simulink model "RollingMill_PLC"  (R2020b)
settings: Solver=ode1be  StartTime=0.0  StopTime=inf  RelTol=1e-3
values from neighbouring files (symbols this model uses):
  sysd_2 = c2d(sysc,0.01)    [Rolling_mill_matlab.m]
libraries: simulink x4, opclib x1
settings Model: Creator=Mehrab  LastModifiedBy=Mehrab
settings DataIOCC: LimitDataPoints=on  SaveFormat=Array  SaveOutput=off  SaveTime=off
settings OptimizationCC: LifeSpan=1
settings HardwareCC: ProdBitPerPointer=32  ProdBitPerSizeT=32  ProdBitPerPtrDiffT=32  ProdWordSize=32  ProdHWDeviceType=Intel->x86-32 (Windows32)
settings RTWCC: Description=Target for ODK capable S7-1500 Controllers based on Simulink Coder  SystemTargetFile=Target_1500S_V4_0_grt.tlc  GenCodeOnly=on  GenerateMakefile=off  TemplateMakefile=Target_1500S_V4_0_grt.tmf  RTWVerbose=off  TargetLang=C++
settings CodeAppCC: MaxIdLength=256
settings STFCustomTargetCC: TargetLangStandard=C++03 (ISO)  ParMdlRefBuildCompliant=on  ConcurrentExecutionCompliant=off  CombineOutputUpdateFcns=on  CPPClassGenCompliant=off  GRTInterface=off  SystemTargetFile=Target_1500S_V4_0_grt.tlc
settings GRTTargetCC: TargetLangStandard=C++03 (ISO)  CompOptLevelCompliant=off  ConcurrentExecutionCompliant=off  MatFileLogging=off  CPPClassGenCompliant=off  UseToolchainInfoCompliant=off  ExtModeStaticAlloc=on  ExtModeMexFile=mwsl_ii_ext_comm_target1500s_v4  ExtModeMexArgs='192.168.3.3' 0 17725 0

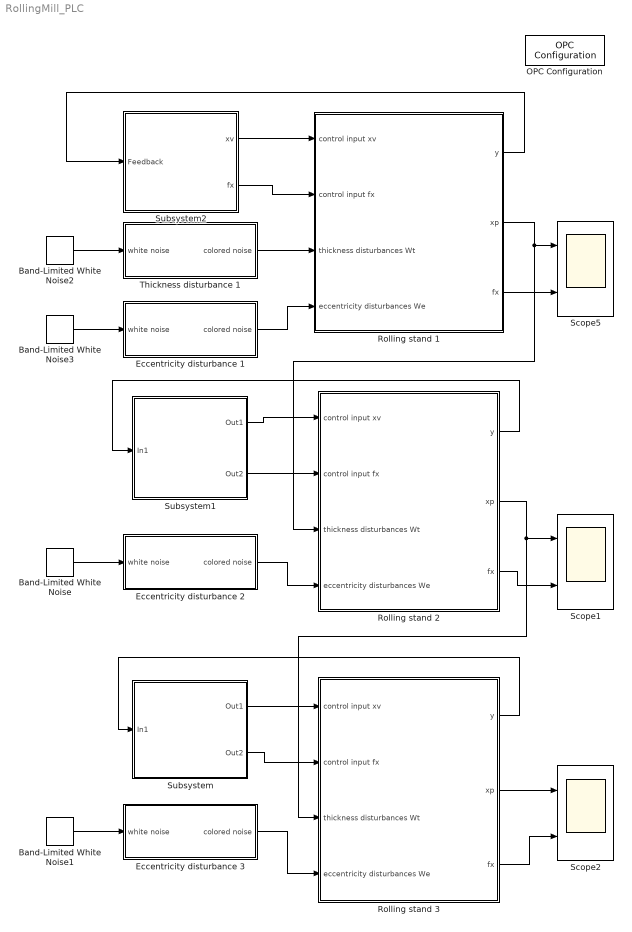
== system RollingMill_PLC ==
  Band-Limited White Noise : simulink/Sources/Band-Limited White Noise  Cov=[0.0001]  Ts=0.01  seed=[21241]
  Band-Limited White Noise1 : simulink/Sources/Band-Limited White Noise  Cov=[0.00001]  Ts=0.01  seed=[63341]
  Band-Limited White Noise2 : simulink/Sources/Band-Limited White Noise  Cov=[15]  Ts=0.01  seed=[23341]
  Band-Limited White Noise3 : simulink/Sources/Band-Limited White Noise  Cov=[0.0001]  Ts=0.01  seed=[65441]
  Eccentricity disturbance 1 : Subsystem
  Eccentricity disturbance 2 : Subsystem
  Eccentricity disturbance 3 : Subsystem
  OPC Configuration : opclib/OPC Configuration  errMissingItems=Error  errReadWrite=Warn  errShutdown=Error  errRTViolation=Warn  rtEnable=on  speedup=1  showLatency=off  beingUsed=on
      settings: SourceProductBaseCode=OT
  Rolling stand 1 : Subsystem
      mask Display:
      | image('$imagefile'); % Use "Edit Image" on toolstrip to change.
      | color('blue');port_label('input', 1, 'xv');
      | port_label('input', 2, 'fx');
      | color('red');port_label('input', 3, 'Wt');
      | port_label('input', 4, 'We');
      | color('black');port_label('output', 1, 'y');
      | port_label('output', 2, 'xp');
      | port_label('output', 3, 'fx');
  Rolling stand 2 : Subsystem
      mask Display:
      | image('$imagefile'); % Use "Edit Image" on toolstrip to change.
      | color('blue');port_label('input', 1, 'xv');
      | port_label('input', 2, 'fx');
      | color('red');port_label('input', 3, 'Wt');
      | port_label('input', 4, 'We');
      | color('black');port_label('output', 1, 'y');
      | port_label('output', 2, 'xp');
      | port_label('output', 3, 'fx');
  Rolling stand 3 : Subsystem
      mask Display:
      | image('$imagefile'); % Use "Edit Image" on toolstrip to change.
      | color('blue');port_label('input', 1, 'xv');
      | port_label('input', 2, 'fx');
      | color('red');port_label('input', 3, 'Wt');
      | port_label('input', 4, 'We');
      | color('black');port_label('output', 1, 'y');
      | port_label('output', 2, 'xp');
      | port_label('output', 3, 'fx');
  Scope1 : Scope  NumInputPorts=2
  Scope2 : Scope  NumInputPorts=2
  Scope5 : Scope  NumInputPorts=2
  Subsystem : Subsystem
      mask Display: image('$imagefile'); % Use "Edit Image" on toolstrip to change.
  Subsystem1 : Subsystem
      mask Display: image('$imagefile'); % Use "Edit Image" on toolstrip to change.
  Subsystem2 : Subsystem
      mask Display: image('$imagefile'); % Use "Edit Image" on toolstrip to change.
  Thickness disturbance 1 : Subsystem
  wires:
  Rolling stand 1/2(xp) -> Scope5/1, Rolling stand 2/3(thickness disturbances Wt)
  Rolling stand 1/3(fx) -> Scope5/2
  Thickness disturbance 1/1(colored noise) -> Rolling stand 1/3(thickness disturbances Wt)
  Band-Limited White Noise3/1 -> Eccentricity disturbance 1/1(white noise)
  Eccentricity disturbance 1/1(colored noise) -> Rolling stand 1/4(eccentricity disturbances We)
  Band-Limited White Noise/1 -> Eccentricity disturbance 2/1(white noise)
  Eccentricity disturbance 2/1(colored noise) -> Rolling stand 2/4(eccentricity disturbances We)
  Rolling stand 2/3(fx) -> Scope1/2
  Rolling stand 3/2(xp) -> Scope2/1
  Rolling stand 3/3(fx) -> Scope2/2
  Eccentricity disturbance 3/1(colored noise) -> Rolling stand 3/4(eccentricity disturbances We)
  Band-Limited White Noise1/1 -> Eccentricity disturbance 3/1(white noise)
  Rolling stand 2/2(xp) -> Scope1/1, Rolling stand 3/3(thickness disturbances Wt)
  Band-Limited White Noise2/1 -> Thickness disturbance 1/1(white noise)
  Rolling stand 3/1(y) -> Subsystem/1(In1)
  Subsystem/1(Out1) -> Rolling stand 3/1(control input xv)
  Subsystem/2(Out2) -> Rolling stand 3/2(control input fx)
  Rolling stand 2/1(y) -> Subsystem1/1(In1)
  Subsystem1/1(Out1) -> Rolling stand 2/1(control input xv)
  Subsystem1/2(Out2) -> Rolling stand 2/2(control input fx)
  Rolling stand 1/1(y) -> Subsystem2/1(Feedback)
  Subsystem2/1(xv) -> Rolling stand 1/1(control input xv)
  Subsystem2/2(fx) -> Rolling stand 1/2(control input fx)

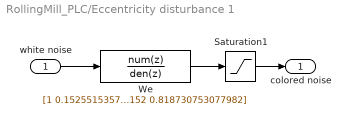
== system RollingMill_PLC/Eccentricity disturbance 1 ==
  white noise : Inport
  Saturation1 : Saturate
  We : DiscreteTransferFcn  Numerator=[1 0.152551535702048 -0.152551535702048]  Denominator=[1 -0.985392246190152 0.818730753077982]
  colored noise : Outport
  wires:
  white noise/1 -> We/1
  We/1 -> Saturation1/1
  Saturation1/1 -> colored noise/1

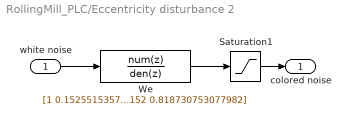
== system RollingMill_PLC/Eccentricity disturbance 2 ==
  white noise : Inport
  Saturation1 : Saturate
  We : DiscreteTransferFcn  Numerator=[1 0.152551535702048 -0.152551535702048]  Denominator=[1 -0.985392246190152 0.818730753077982]
  colored noise : Outport
  wires:
  Saturation1/1 -> colored noise/1
  We/1 -> Saturation1/1
  white noise/1 -> We/1

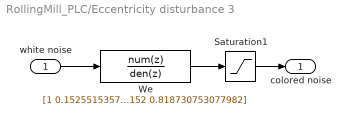
== system RollingMill_PLC/Eccentricity disturbance 3 ==
  white noise : Inport
  Saturation1 : Saturate  UpperLimit=0.2  LowerLimit=-0.2
  We : DiscreteTransferFcn  Numerator=[1 0.152551535702048 -0.152551535702048]  Denominator=[1 -0.985392246190152 0.818730753077982]
  colored noise : Outport
  wires:
  white noise/1 -> We/1
  We/1 -> Saturation1/1
  Saturation1/1 -> colored noise/1

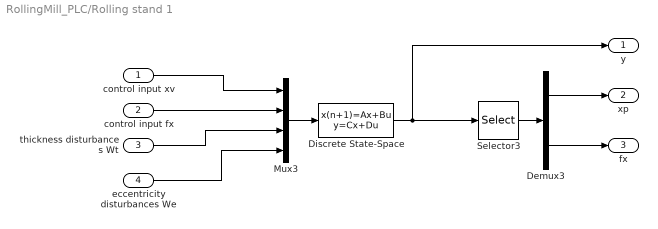
== system RollingMill_PLC/Rolling stand 1 ==
  control input xv : Inport
  control input fx : Inport  Port=2
  thickness disturbances Wt : Inport  Port=3
  eccentricity disturbances We : Inport  Port=4
  Demux3 : Demux  Outputs=2
  Discrete State-Space : DiscreteStateSpace  A=sysd_2.A  B=sysd_2.B  C=sysd_2.C  D=sysd_2.D  SampleTime=-1
  Mux3 : Mux
  Selector3 : Selector  InputPortWidth=5  IndexOptions=Index vector (dialog)  Indices=[3 5]  OutputSizes=1
  y : Outport
  xp : Outport  Port=2
  fx : Outport  Port=3
  wires:
  Selector3/1 -> Demux3/1
  eccentricity disturbances We/1 -> Mux3/4
  Discrete State-Space/1 -> y/1, Selector3/1
  Mux3/1 -> Discrete State-Space/1
  control input fx/1 -> Mux3/2
  thickness disturbances Wt/1 -> Mux3/3
  Demux3/1 -> xp/1
  control input xv/1 -> Mux3/1
  Demux3/2 -> fx/1

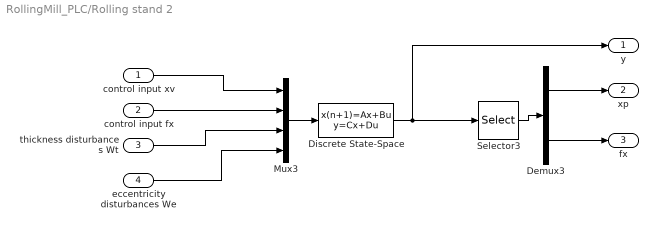
== system RollingMill_PLC/Rolling stand 2 ==
  control input xv : Inport
  control input fx : Inport  Port=2
  thickness disturbances Wt : Inport  Port=3
  eccentricity disturbances We : Inport  Port=4
  Demux3 : Demux  Outputs=2
  Discrete State-Space : DiscreteStateSpace  A=sysd_2.A  B=sysd_2.B  C=sysd_2.C  D=sysd_2.D  SampleTime=-1
  Mux3 : Mux
  Selector3 : Selector  InputPortWidth=5  IndexOptions=Index vector (dialog)  Indices=[3 5]  OutputSizes=1
  y : Outport
  xp : Outport  Port=2
  fx : Outport  Port=3
  wires:
  Demux3/2 -> fx/1
  control input xv/1 -> Mux3/1
  Demux3/1 -> xp/1
  thickness disturbances Wt/1 -> Mux3/3
  control input fx/1 -> Mux3/2
  Mux3/1 -> Discrete State-Space/1
  Discrete State-Space/1 -> Selector3/1, y/1
  eccentricity disturbances We/1 -> Mux3/4
  Selector3/1 -> Demux3/1

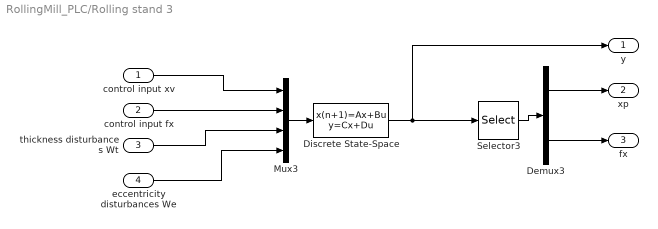
== system RollingMill_PLC/Rolling stand 3 ==
  control input xv : Inport
  control input fx : Inport  Port=2
  thickness disturbances Wt : Inport  Port=3
  eccentricity disturbances We : Inport  Port=4
  Demux3 : Demux  Outputs=2
  Discrete State-Space : DiscreteStateSpace  A=sysd_2.A  B=sysd_2.B  C=sysd_2.C  D=sysd_2.D  SampleTime=-1
  Mux3 : Mux
  Selector3 : Selector  InputPortWidth=5  IndexOptions=Index vector (dialog)  Indices=[3 5]  OutputSizes=1
  y : Outport
  xp : Outport  Port=2
  fx : Outport  Port=3
  wires:
  Selector3/1 -> Demux3/1
  eccentricity disturbances We/1 -> Mux3/4
  Discrete State-Space/1 -> y/1, Selector3/1
  Mux3/1 -> Discrete State-Space/1
  control input fx/1 -> Mux3/2
  thickness disturbances Wt/1 -> Mux3/3
  Demux3/1 -> xp/1
  control input xv/1 -> Mux3/1
  Demux3/2 -> fx/1

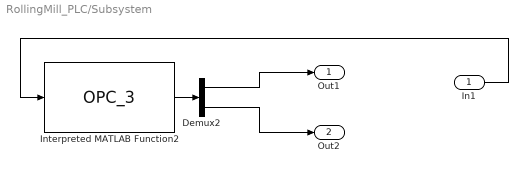
== system RollingMill_PLC/Subsystem ==
  In1 : Inport
  Demux2 : Demux  Outputs=2
  Interpreted MATLAB Function2 : MATLABFcn  MATLABFcn=OPC_3  OutputDimensions=2
  Out1 : Outport
  Out2 : Outport  Port=2
  wires:
  Interpreted MATLAB Function2/1 -> Demux2/1
  In1/1 -> Interpreted MATLAB Function2/1
  Demux2/1 -> Out1/1
  Demux2/2 -> Out2/1

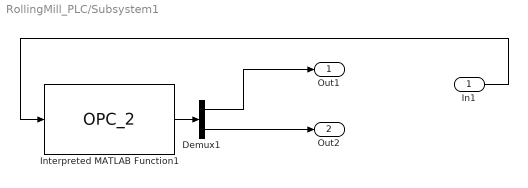
== system RollingMill_PLC/Subsystem1 ==
  In1 : Inport
  Demux1 : Demux  Outputs=2
  Interpreted MATLAB Function1 : MATLABFcn  MATLABFcn=OPC_2  OutputDimensions=2
  Out1 : Outport
  Out2 : Outport  Port=2
  wires:
  Interpreted MATLAB Function1/1 -> Demux1/1
  Demux1/2 -> Out2/1
  Demux1/1 -> Out1/1
  In1/1 -> Interpreted MATLAB Function1/1

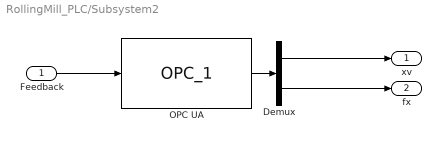
== system RollingMill_PLC/Subsystem2 ==
  Feedback : Inport
  Demux : Demux  Outputs=2
  OPC UA : MATLABFcn  MATLABFcn=OPC_1  OutputDimensions=2
  xv : Outport
  fx : Outport  Port=2
  wires:
  OPC UA/1 -> Demux/1
  Demux/2 -> fx/1
  Feedback/1 -> OPC UA/1
  Demux/1 -> xv/1

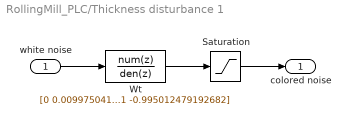
== system RollingMill_PLC/Thickness disturbance 1 ==
  white noise : Inport
  Saturation : Saturate  UpperLimit=4  LowerLimit=-4
  Wt : DiscreteTransferFcn  Numerator=[0 0.009975041614635]  Denominator=[1 -0.995012479192682]
  colored noise : Outport
  wires:
  white noise/1 -> Wt/1
  Saturation/1 -> colored noise/1
  Wt/1 -> Saturation/1
